simulink library "calcTangentRollAngle_ul"  (R2020a)
settings: Solver=VariableStepAuto  StartTime=0.0  StopTime=10.0  RelTol=1e-3
libraries: angleBtwVecs_ul x1
settings Model: Creator=Ayaz  LastModifiedBy=Ayaz

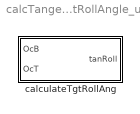
== system calcTangentRollAngle_ul ==
  calculateTgtRollAng : Subsystem

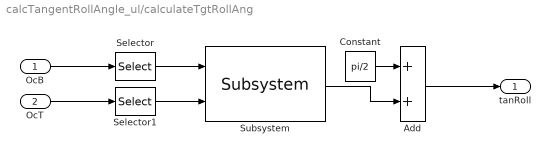
== system calcTangentRollAngle_ul/calculateTgtRollAng ==
  OcB : Inport
  OcT : Inport  Port=2
  Add : Sum
  Constant : Constant  Value=pi/2
  Selector : Selector  NumberOfDimensions=2  InputPortWidth=3  IndexOptions=Index vector (dialog),Index vector (dialog)  Indices=[1 2 3],2  OutputSizes=1,1
  Selector1 : Selector  NumberOfDimensions=2  InputPortWidth=3  IndexOptions=Index vector (dialog),Index vector (dialog)  Indices=[1 2 3],3  OutputSizes=1,1
  Subsystem : angleBtwVecs_ul/Subsystem  SystemSampleTime=-1  Latency=0  AutoFrameSizeCalculation=off
  tanRoll : Outport
  wires:
  OcB/1 -> Selector/1
  OcT/1 -> Selector1/1
  Subsystem/1 -> Add/2
  Selector/1 -> Subsystem/1
  Selector1/1 -> Subsystem/2
  Constant/1 -> Add/1
  Add/1 -> tanRoll/1
